simulink model "chirp_test"  (R2018a)
settings: Solver=VariableStepAuto  StartTime=0.0  StopTime=param_simtime  RelTol=1e-3
values from neighbouring files (symbols this model uses):
  param_f_res = 0.5    [plot_chirp.m]
libraries: dspsrcs4 x1, simulink x1
settings Model: Creator=tim  LastModifiedBy=Tim

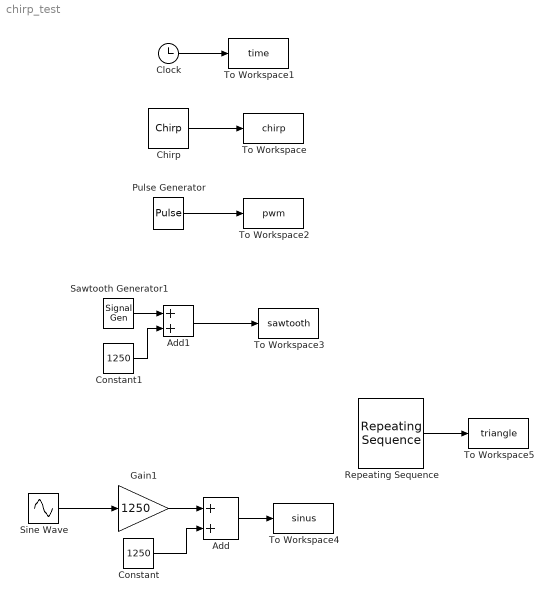
== system chirp_test ==
  Add : Sum
  Add1 : Sum
  Chirp : dspsrcs4/Chirp  sweep=Linear  mode=Unidirectional  f0=0  f1=param_simtime  t1=param_simtime  Tsweep=param_simtime  phase=0  Ts=1/1000  spf=1  datatype=Double  OutputFrames=off
      settings: SourceProductName=DSP System Toolbox
  Clock : Clock
  Constant : Constant  Value=1250
  Constant1 : Constant  Value=1250
  Gain1 : Gain  Gain=1250
  Pulse Generator : DiscretePulseGenerator  PulseType=Time based  Amplitude=2500  Period=1/param_f_res  PulseWidth=50
  Repeating Sequence : simulink/Sources/Repeating Sequence  rep_seq_t=[0 (1/(2*param_f_res)) 1/param_f_res]  rep_seq_y=[0 2500 0]
  Sawtooth Generator1 : SignalGenerator  WaveForm=sawtooth  Amplitude=1250  Frequency=param_f_res*5  Units=rad/sec
  Sine Wave : Sin  Frequency=param_f_res*5  SampleTime=0
  To Workspace : ToWorkspace  VariableName=chirp  SampleTime=-1
      settings: Save2DSignal=2-D array (concatenate along first dimension)
  To Workspace1 : ToWorkspace  VariableName=time  SampleTime=-1
      settings: Save2DSignal=2-D array (concatenate along first dimension)
  To Workspace2 : ToWorkspace  VariableName=pwm  SampleTime=-1
      settings: Save2DSignal=2-D array (concatenate along first dimension)
  To Workspace3 : ToWorkspace  VariableName=sawtooth  SampleTime=-1
      settings: Save2DSignal=2-D array (concatenate along first dimension)
  To Workspace4 : ToWorkspace  VariableName=sinus  SampleTime=-1
      settings: Save2DSignal=2-D array (concatenate along first dimension)
  To Workspace5 : ToWorkspace  VariableName=triangle  SampleTime=-1
      settings: Save2DSignal=2-D array (concatenate along first dimension)
  wires:
  Chirp/1 -> To Workspace/1
  Clock/1 -> To Workspace1/1
  Pulse Generator/1 -> To Workspace2/1
  Add1/1 -> To Workspace3/1
  Constant/1 -> Add/2
  Sine Wave/1 -> Gain1/1
  Gain1/1 -> Add/1
  Add/1 -> To Workspace4/1
  Repeating Sequence/1 -> To Workspace5/1
  Constant1/1 -> Add1/2
  Sawtooth Generator1/1 -> Add1/1
